simulink model "sim_lab6_recapitulare"  (R2024b)
settings: Solver=VariableStepAuto  StartTime=0.0  StopTime=0.3  RelTol=1e-3
values from neighbouring files (symbols this model uses):
  A = [-Ra/La, -K/La; K/J, 0;]    [Lab6.m]    (also in Lab6_recapitulare.m)
  B = [1/La, 0; 0, -1/J]    [Lab6.m]    (also in Lab6_recapitulare.m)
  C = [1, 0; 0, 1]    [Lab6.m]    (also in Lab6_recapitulare.m)
  D = [0, 0; 0, 0]    [Lab6.m]    (also in Lab6_recapitulare.m)
  Ts = 0.001    [Lab6.m]    (also in Lab6_recapitulare.m)
settings Model: Creator=akopo  LastModifiedBy=akopo

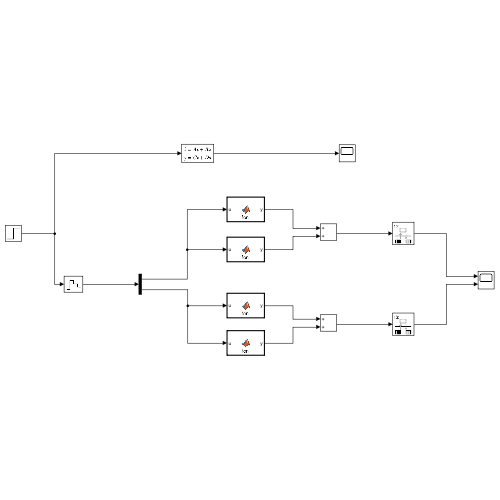
[thumbnail: Simulink's stored preview of the top-level diagram]
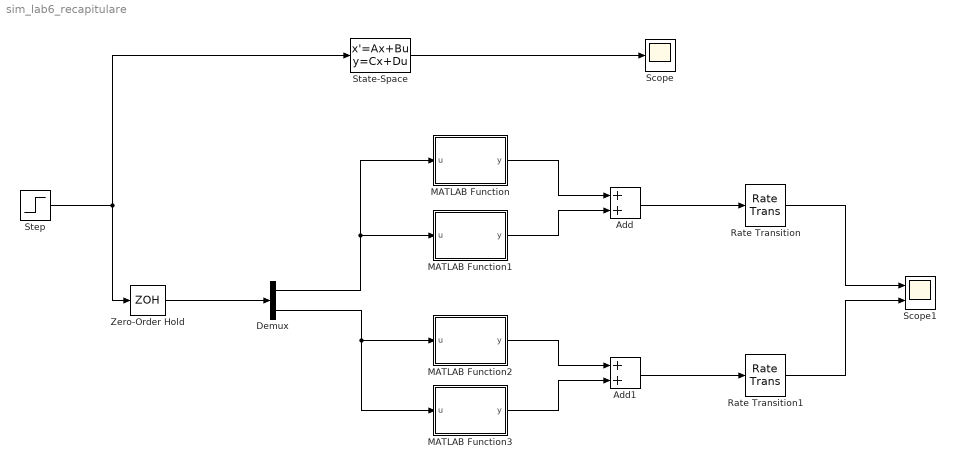
== system sim_lab6_recapitulare ==
  Add : Sum
  Add1 : Sum
  Demux : Demux  Outputs=2
  MATLAB Function : MATLAB Function  TreatAsAtomicUnit=on
  MATLAB Function1 : MATLAB Function  TreatAsAtomicUnit=on
  MATLAB Function2 : MATLAB Function  TreatAsAtomicUnit=on
  MATLAB Function3 : MATLAB Function  TreatAsAtomicUnit=on
  Rate Transition : RateTransition
  Rate Transition1 : RateTransition
  Scope : Scope
  Scope1 : Scope  NumInputPorts=2
  State-Space : StateSpace  A=A  B=B  C=C  D=D  InitialCondition=0
  Step : Step  Time=0  Before=[0, 0]  After=[25, 0]  SampleTime=Ts
  Zero-Order Hold : ZeroOrderHold  SampleTime=-1
  wires:
  State-Space/1 -> Scope/1
  Step/1 -> State-Space/1, Zero-Order Hold/1
  Zero-Order Hold/1 -> Demux/1
  Demux/1 -> MATLAB Function/1(u), MATLAB Function1/1(u)
  Demux/2 -> MATLAB Function3/1(u), MATLAB Function2/1(u)
  MATLAB Function/1(y) -> Add/1
  MATLAB Function1/1(y) -> Add/2
  Add/1 -> Rate Transition/1
  Rate Transition/1 -> Scope1/1
  Rate Transition1/1 -> Scope1/2
  Add1/1 -> Rate Transition1/1
  MATLAB Function2/1(y) -> Add1/1
  MATLAB Function3/1(y) -> Add1/2

== matlab function sim_lab6_recapitulare/MATLAB Function ==
  data: u input; y output
function y = fcn(u)

persistent y1 y2 u1 u2;

if isempty(y2)
    y2 = 0;
end

if isempty(y1)
    y1 = 0;
end

if isempty(u1)
    u1 = 0;
end

if isempty(u2)
    u2 = 0;
end

a = 0.346;
b = -0.346;
c = -1.41;
d = 0.4421;

y = - c * y1 - d * y2 + a * u1 + b * u2;

u2 = u1;
u1 = u;
y2 = y1;
y1 = y;

== matlab function sim_lab6_recapitulare/MATLAB Function2 ==
  data: u input; y output
function y = fcn(u)

persistent y1 y2 u1 u2;

if isempty(y2)
    y2 = 0;
end

if isempty(y1)
    y1 = 0;
end

if isempty(u1)
    u1 = 0;
end

if isempty(u2)
    u2 = 0;
end

a = 0.2791;
b = 0.2128;
c = -1.41;
d = 0.4421;

y = - c * y1 - d * y2 + a * u1 + b * u2;

u2 = u1;
u1 = u;
y2 = y1;
y1 = y;

== matlab function sim_lab6_recapitulare/MATLAB Function3 ==
  data: u input; y output
function y = fcn(u)

persistent y1 y2 u1 u2;

if isempty(y2)
    y2 = 0;
end

if isempty(y1)
    y1 = 0;
end

if isempty(u1)
    u1 = 0;
end

if isempty(u2)
    u2 = 0;
end

a = -21.65;
b = 9.537;
c = -1.41;
d = 0.4421;

y = -c * y1 - d * y2 + a * u1 + b * u2;

u2 = u1;
u1 = u;
y2 = y1;
y1 = y;

== matlab function sim_lab6_recapitulare/MATLAB Function1 ==
  data: u input; y output
function y = fcn(u)

persistent y1 y2 u1 u2;

if isempty(y2)
    y2 = 0;
end

if isempty(y1)
    y1 = 0;
end

if isempty(u1)
    u1 = 0;
end

if isempty(u2)
    u2 = 0;
end

a = 0.2791;
b = 0.2128;
c = -1.41;
d = 0.4421;

y = -c * y1 - d * y2 + a * u1 + b * u2;

u2 = u1;
u1 = u;
y2 = y1;
y1 = y;
